simulink model "encode"  (R2024b)
settings: Solver=FixedStepAuto  StartTime=0.0  StopTime=inf  FixedStep=0.01  RelTol=1e-3  EnableMultiTasking=on
libraries: simulink x6, stm32f4xxblockslib x5, stm32g4xxblockslib x3
settings Model: STM32="{\"EncoderBlockForG4\":[{\"ID\":\"encode:1\"},{\"ID\":\"encode:52\"},{\"ID\":\"encode:72\"}],\"DigitalPortRead\":[{\"ID\":\"encode:8\"},{\"ID\":\"encode:7\"},{\"ID\":\"encode:60\"},{\"ID\":\"encode:80\"},{\"ID\":\"encode:25\"}]}"  Creator=A1nz_01  LastModifiedBy=A1nz_01
settings OptimizationCC: DefaultParameterBehavior=Inlined  EnhancedBackFolding=on  PassReuseOutputArgsAs=Individual arguments  ZeroExternalMemoryAtStartup=off  ZeroInternalMemoryAtStartup=off  MaxStackSize=512  OptimizeBlockOrder=speed  DifferentSizesBufferReuse=on  OptimizationCustomize=off  EfficientTunableParamExpr=on
settings DebuggingCC: ParameterTunabilityLossMsg=error
settings HardwareCC: ProdBitPerPointer=32  ProdBitPerSizeT=32  ProdBitPerPtrDiffT=32  ProdLargestAtomicInteger=Long  ProdLargestAtomicFloat=Double  ProdWordSize=32  ProdLongLongMode=on  ProdHWDeviceType=ARM Compatible->ARM Cortex-M
settings SFSimCC: MATLABDynamicMemAlloc=off
settings RTWCC: Description=Embedded Coder  SystemTargetFile=ert.tlc  HardwareBoard=STM32G4xx Based  TemplateMakefile=ert_default_tmf  Toolchain=GNU Tools for ARM Embedded Processors
settings CodeAppCC: ForceParamTrailComments=on  IgnoreCustomStorageClasses=off  OperatorAnnotations=on  SimulinkDataObjDesc=on  SFDataObjDesc=on  InsertBlockDesc=on
settings ERTTargetCC: TargetLangStandard=C99 (ISO)  CodeReplacementLibrary=ARM Cortex-M  ExtModeTransport=3  ExtModeStaticAlloc=on  ExtModeStaticAllocSize=2048  ExtModeMexFile=ext_xcp  ExtModeIntrfLevel=Level2 - Open

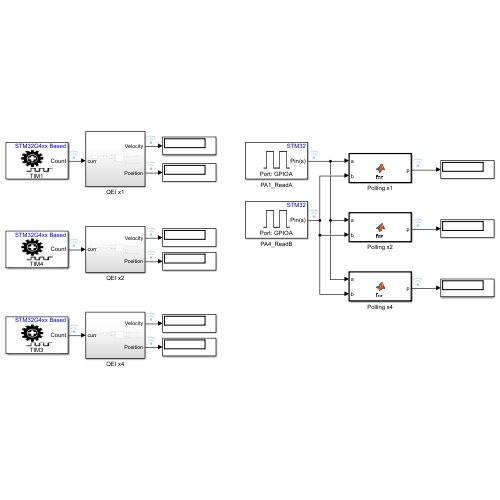
[thumbnail: Simulink's stored preview of the top-level diagram]
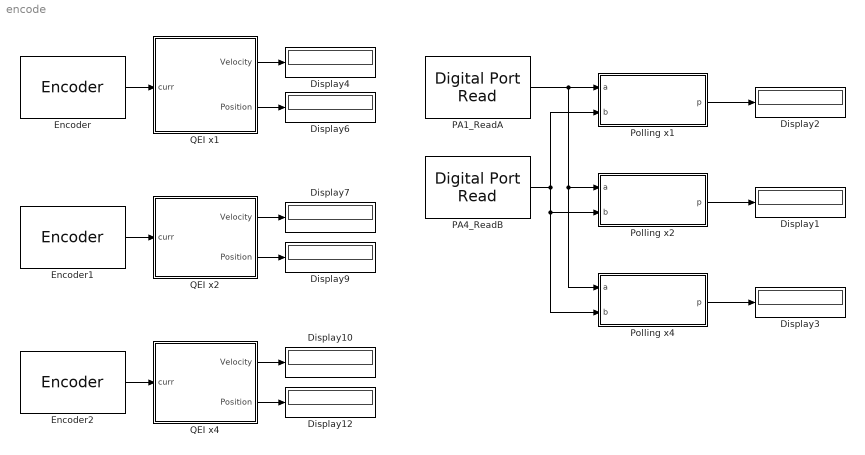
== system encode ==
  Display{1..4,6..7,9..10,12} (9 alike) : Display
  Encoder : stm32g4xxblockslib/Encoder  TimerModule=TIM1  EnableResetInput=off  OutputCountAfterFirstIndex=off  OutputValidIndex=off  OutputDirection=off  OutputStatus=off  SampleTime=-1
  Encoder1 : stm32g4xxblockslib/Encoder  TimerModule=TIM4  EnableResetInput=off  OutputCountAfterFirstIndex=off  OutputValidIndex=off  OutputDirection=off  OutputStatus=off  SampleTime=-1
  Encoder2 : stm32g4xxblockslib/Encoder  TimerModule=TIM3  EnableResetInput=off  OutputCountAfterFirstIndex=off  OutputValidIndex=off  OutputDirection=off  OutputStatus=off  SampleTime=-1
  PA1_ReadA : stm32f4xxblockslib/Digital Port Read  PortName=GPIOA  PinNumber=[1]  ReadOperation=on  IOAsArray=on  SampleTime=-1  EnableSimPort=off  hoistedMaskSrc=ECSoC/ECSimCodegen/Digital Port Read
      settings: LibrarySourceBlock=stm32g4xxblockslib/Digital Port Read
  PA4_ReadB : stm32f4xxblockslib/Digital Port Read  PortName=GPIOA  PinNumber=[4]  ReadOperation=on  IOAsArray=on  SampleTime=-1  EnableSimPort=off  hoistedMaskSrc=ECSoC/ECSimCodegen/Digital Port Read
      settings: LibrarySourceBlock=stm32g4xxblockslib/Digital Port Read
  Polling x1 : MATLAB Function  TreatAsAtomicUnit=on
  Polling x2 : MATLAB Function  TreatAsAtomicUnit=on
  Polling x4 : MATLAB Function  TreatAsAtomicUnit=on
  QEI x1 : Subsystem
  QEI x2 : Subsystem
  QEI x4 : Subsystem
  wires:
  PA4_ReadB/1 -> Polling x2/2(b), Polling x4/2(b), Polling x1/2(b)
  PA1_ReadA/1 -> Polling x4/1(a), Polling x2/1(a), Polling x1/1(a)
  Encoder/1 -> QEI x1/1(curr)
  QEI x1/1(Velocity) -> Display4/1
  QEI x1/2(Position) -> Display6/1
  QEI x2/2(Position) -> Display9/1
  QEI x2/1(Velocity) -> Display7/1
  Encoder1/1 -> QEI x2/1(curr)
  QEI x4/2(Position) -> Display12/1
  QEI x4/1(Velocity) -> Display10/1
  Encoder2/1 -> QEI x4/1(curr)
  Polling x1/1(p) -> Display2/1
  Polling x2/1(p) -> Display1/1
  Polling x4/1(p) -> Display3/1

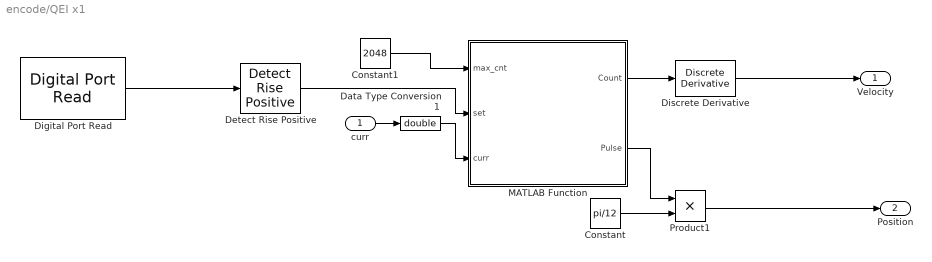
== system encode/QEI x1 ==
  curr : Inport
  Constant : Constant  Value=pi/12
  Constant1 : Constant  Value=2048
  Data Type Conversion1 : DataTypeConversion  OutDataTypeStr=double  SaturateOnIntegerOverflow=off  RndMeth=Floor
  Detect Rise Positive : simulink/Logic and Bit Operations/Detect Rise Positive  vinit=0  OutDataTypeStr=boolean
  Digital Port Read : stm32f4xxblockslib/Digital Port Read  PortName=GPIOC  PinNumber=[13]  ReadOperation=on  IOAsArray=on  SampleTime=-1  EnableSimPort=off  hoistedMaskSrc=ECSoC/ECSimCodegen/Digital Port Read
      settings: LibrarySourceBlock=stm32g4xxblockslib/Digital Port Read
  Discrete Derivative : simulink/Discrete/Discrete Derivative  gainval=1.0  ICPrevScaledInput=0.0  OutMin=[]  OutMax=[]  OutDataType=fixdt(1, 16)  OutScaling=2^-10  DoSatur=off
  MATLAB Function : MATLAB Function  TreatAsAtomicUnit=on
  Product1 : Product
  Velocity : Outport
  Position : Outport  Port=2
  wires:
  Digital Port Read/1 -> Detect Rise Positive/1
  Detect Rise Positive/1 -> MATLAB Function/2(set)
  Data Type Conversion1/1 -> MATLAB Function/3(curr)
  curr/1 -> Data Type Conversion1/1
  MATLAB Function/1(Count) -> Discrete Derivative/1
  Discrete Derivative/1 -> Velocity/1
  MATLAB Function/2(Pulse) -> Product1/1
  Constant/1 -> Product1/2
  Product1/1 -> Position/1
  Constant1/1 -> MATLAB Function/1(max_cnt)

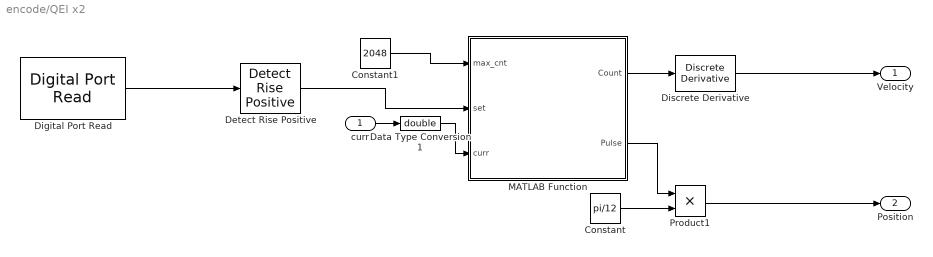
== system encode/QEI x2 ==
  curr : Inport
  Constant : Constant  Value=pi/12
  Constant1 : Constant  Value=2048
  Data Type Conversion1 : DataTypeConversion  OutDataTypeStr=double  SaturateOnIntegerOverflow=off  RndMeth=Floor
  Detect Rise Positive : simulink/Logic and Bit Operations/Detect Rise Positive  vinit=0  OutDataTypeStr=boolean
  Digital Port Read : stm32f4xxblockslib/Digital Port Read  PortName=GPIOC  PinNumber=[13]  ReadOperation=on  IOAsArray=on  SampleTime=-1  EnableSimPort=off  hoistedMaskSrc=ECSoC/ECSimCodegen/Digital Port Read
  Discrete Derivative : simulink/Discrete/Discrete Derivative  gainval=1.0  ICPrevScaledInput=0.0  OutMin=[]  OutMax=[]  OutDataType=fixdt(1, 16)  OutScaling=2^-10  DoSatur=off
  MATLAB Function : MATLAB Function  TreatAsAtomicUnit=on
  Product1 : Product
  Velocity : Outport
  Position : Outport  Port=2
  wires:
  Digital Port Read/1 -> Detect Rise Positive/1
  Detect Rise Positive/1 -> MATLAB Function/2(set)
  Data Type Conversion1/1 -> MATLAB Function/3(curr)
  curr/1 -> Data Type Conversion1/1
  MATLAB Function/1(Count) -> Discrete Derivative/1
  Discrete Derivative/1 -> Velocity/1
  MATLAB Function/2(Pulse) -> Product1/1
  Constant/1 -> Product1/2
  Product1/1 -> Position/1
  Constant1/1 -> MATLAB Function/1(max_cnt)

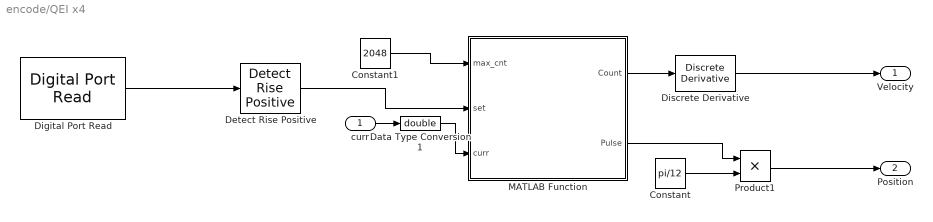
== system encode/QEI x4 ==
  curr : Inport
  Constant : Constant  Value=pi/12
  Constant1 : Constant  Value=2048
  Data Type Conversion1 : DataTypeConversion  OutDataTypeStr=double  SaturateOnIntegerOverflow=off  RndMeth=Floor
  Detect Rise Positive : simulink/Logic and Bit Operations/Detect Rise Positive  vinit=0  OutDataTypeStr=boolean
  Digital Port Read : stm32f4xxblockslib/Digital Port Read  PortName=GPIOC  PinNumber=[13]  ReadOperation=on  IOAsArray=on  SampleTime=-1  EnableSimPort=off  hoistedMaskSrc=ECSoC/ECSimCodegen/Digital Port Read
  Discrete Derivative : simulink/Discrete/Discrete Derivative  gainval=1.0  ICPrevScaledInput=0.0  OutMin=[]  OutMax=[]  OutDataType=fixdt(1, 16)  OutScaling=2^-10  DoSatur=off
  MATLAB Function : MATLAB Function  TreatAsAtomicUnit=on
  Product1 : Product
  Velocity : Outport
  Position : Outport  Port=2
  wires:
  Digital Port Read/1 -> Detect Rise Positive/1
  Detect Rise Positive/1 -> MATLAB Function/2(set)
  Data Type Conversion1/1 -> MATLAB Function/3(curr)
  curr/1 -> Data Type Conversion1/1
  MATLAB Function/1(Count) -> Discrete Derivative/1
  Discrete Derivative/1 -> Velocity/1
  MATLAB Function/2(Pulse) -> Product1/1
  Constant/1 -> Product1/2
  Product1/1 -> Position/1
  Constant1/1 -> MATLAB Function/1(max_cnt)

== matlab function encode/Polling x2 ==
  data: a input; p output; b input
function p = fcn(a,b)
    persistent pos;
    persistent trig;
    if isempty(trig)
        trig = 1;
        pos = 0;
    end
    if a-b == -1 && trig
        pos = pos + 1;
        trig = 2;
    elseif a-b == 1 && trig
        pos = pos -1;
        trig = 2;
    end

    if a == 0 && b == 0 
        trig = 0;
    end

    if a-b == 1 && trig == 0
        pos = pos + 1;
        trig = -1;
    elseif a-b == -1 && trig == 0
        pos = pos -1;
        trig = 1;
    end

    if a == 1 && b == 1
        trig = 1;
    end
    p = pos;
end

== matlab function encode/Polling x1 ==
  data: a input; p output; b input
function p = fcn(a,b)
    persistent pos;
    persistent trig;
    if isempty(trig)
        trig = 1;
        pos = 0;
    end
    if a-b == -1 && trig
        pos = pos + 1;
        trig = 0;
    elseif a-b == 1 && trig
        pos = pos -1;
        trig = 0;
    end

    if a == 1 && b == 1
        trig = 1;
    end
    p = pos;
end

== matlab function encode/Polling x4 ==
  data: a input; p output; b input
function p = fcn(a,b)
    persistent pos;
    persistent trigA;
    persistent trigB;
    if isempty(trigA)
        trigA = 1;
        trigB = 1;
        pos = 0;
    end
    if a-b == -1 && trigA
        pos = pos + 1;
        trigA = 2;
    elseif a-b == 1 && trigA
        pos = pos -1;
        trigA = 2;
    end


    if a-b == -1 && trigA == 0
        pos = pos + 1;
        trigA = -1;
    elseif a-b == 1 && trigA == 0
        pos = pos -1;
        trigA = -1;
    end


    if b-a == 1 && trigB
        pos = pos + 1;
        trigB = 2;
    elseif b-a == -1 && trigB
        pos = pos - 1;
        trigB = 2;
    end

    if b-a == 1 && trigB == 0
        pos = pos + 1;
        trigB = -1;
    elseif b-a == -1 && trigB == 0
        pos = pos - 1;
        trigB = -1;
    end

    if a == 0 && b == 0
        trigA = 0;
        trigB = 0;
    end

    if a == 1 && b == 1
        trigA = 1;
        trigB = 1;
    end
    p = pos;
end

== matlab function encode/QEI x1/MATLAB Function ==
  data: max_cnt input; Count output; Pulse output; set input; curr input
function [Count,Pulse] = fcn(max_cnt,set,curr)
    persistent prev;
    persistent homing;
    persistent pos;

    if isempty(prev)
        prev = curr;
        homing = 0;
        pos = 0;
    end

    delta = curr - prev;

    if delta <= -1*(max_cnt/2)
        delta = delta + max_cnt + 1;
    elseif delta >= max_cnt/2
        delta = delta -max_cnt - 1;
    end

    if set
        homing = pos;
    end

    pos = pos + delta;
    Count = pos - homing;
    prev = curr;

    Pulse = Count;

end

== matlab function encode/QEI x2/MATLAB Function ==
  data: max_cnt input; Count output; Pulse output; set input; curr input
function [Count,Pulse] = fcn(max_cnt,set,curr)
    persistent prev;
    persistent homing;
    persistent pos;

    if isempty(prev)
        prev = curr;
        homing = 0;
        pos = 0;
    end

    delta = curr - prev;

    if delta <= -1*(max_cnt/2)
        delta = delta + max_cnt + 1;
    elseif delta >= max_cnt/2
        delta = delta -max_cnt - 1;
    end

    if set
        homing = pos;
    end

    pos = pos + delta;
    Count = pos - homing;
    prev = curr;

    Pulse = Count;

end

== matlab function encode/QEI x4/MATLAB Function ==
  data: max_cnt input; Count output; Pulse output; set input; curr input
function [Count,Pulse] = fcn(max_cnt,set,curr)
    persistent prev;
    persistent homing;
    persistent pos;

    if isempty(prev)
        prev = curr;
        homing = 0;
        pos = 0;
    end

    delta = curr - prev;

    if delta <= -1*(max_cnt/2)
        delta = delta + max_cnt + 1;
    elseif delta >= max_cnt/2
        delta = delta -max_cnt - 1;
    end

    if set
        homing = pos;
    end

    pos = pos + delta;
    Count = pos - homing;
    prev = curr;

    Pulse = Count;

end
